simulink model "Wahadlo_final_2015a_2015a"  (R2019a)
settings: Solver=ode5  StartTime=0.0  StopTime=99999  FixedStep=0.01  RelTol=1e-3  AbsTol=1e-6
values from neighbouring files (symbols this model uses):
  K_later = [-K(1) -K(2) K(3)/3 K(4)/3]    [jacobian_calc.m]    (also in linearyzacja.m)
  k_soft_landing = 12    [init.m]
  K_stab = [-K(1) -K(2) K(3)/3 K(4)/3]    [jacobian_calc.m]    (also in linearyzacja.m)
  l = 0.2097    [init.m]    (also in linearyzacja.m = 0.107)
  relay = 0.4    [init.m]
undefined symbols (not defined in the file or in its folder): RTDAC4PCIBaseAddress, sigbuilder_block
settings Model: SimulationMode=external  ExtModeTrigDuration=60000  ExtModeTrigLevel=0.400000  Creator=jims  LastModifiedBy=Radosław
settings SolverCC: AutoScaleAbsTol=off
settings DataIOCC: ExternalInput=[]  InitialState=[]  MaxDataPoints=5000  SaveFormat=Array  SignalLoggingSaveFormat=ModelDataLogs  SaveOutput=off  SaveTime=off  ReturnWorkspaceOutputs=off  SignalLoggingName=sigsOut
settings OptimizationCC: BooleanDataType=off  ExpressionDepthLimit=2147483647  InitFltsAndDblsToZero=on  LifeSpan=inf
settings DebuggingCC: SaveWithParameterizedLinksMsg=none  UnderspecifiedInitializationDetection=Classic  MergeDetectMultiDrivingBlocksExec=none  SignalResolutionControl=TryResolveAllWithWarning  MultiTaskDSMMsg=warning  MultiTaskCondExecSysMsg=none  IntegerOverflowMsg=none  FcnCallInpInsideContextMsg=warning  StateNameClashWarn=warning  SFUnexpectedBacktrackingDiag=warning  SFNoUnconditionalDefaultTransitionDiag=warning  SFExecutionAtInitializationDiag=none  IntegerSaturationMsg=none  ArithmeticOperatorsInVariantConditions=warning
settings HardwareCC: ProdBitPerLong=64  ProdLargestAtomicFloat=None  ProdHWDeviceType=Intel->x86-64  TargetBitPerLong=64  TargetBitPerPointer=64  TargetIntDivRoundTo=Zero  TargetEndianess=LittleEndian  TargetWordSize=64  TargetHWDeviceType=Intel->x86-64
settings ModelReferenceCC: PropagateSignalLabelsOutOfModel=off
settings SFSimCC: SimUseLocalCustomCode=off
settings RTWCC: Description=Real-Time Windows Target  SystemTargetFile=rtwin.tlc  TemplateMakefile=RTDAC_win.tmf  RTWUseLocalCustomCode=off
settings CodeAppCC: StateflowObjectComments=on
settings TargetCC: TargetFcnLib=ansi_tfl_tmw.mat  TargetPreCompLibLocation=C:\Program Files\MATLAB\R2015aSP1\toolbox\sldrt\lib\win64  ModelReferenceCompliant=off  CompOptLevelCompliant=off  PreserveStateflowLocalDataDimensions=off
settings ConfigComp: CovMetricSettings=dw  CovHtmlReporting=on  CovSaveCumulativeToWorkspaceVar=on  CovSaveSingleToWorkspaceVar=on  CovExternalEMLEnable=off

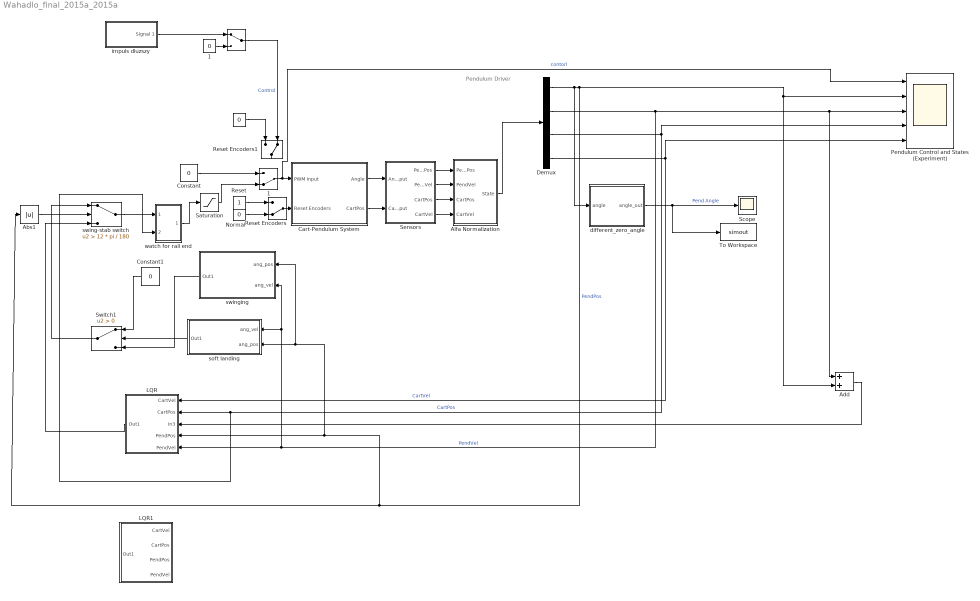
== system Wahadlo_final_2015a_2015a ==
  note: Pendulum
      | Driver
  " " : ManualSwitch
  " " : Constant  Value=0
  " 1" : Constant  Value=0
  " 1" : ManualSwitch  CurrentSetting=0
  Abs1 : Abs
  Add : Sum
  Alfa Normalization : Subsystem  mask(Choose mode:){pos=Inverted Pendulum}
      mask prompts: pos "Choose mode:"
      mask TypeOptions pos: Inverted Pendulum | Crane Controller
  Cart-Pendulum System : Subsystem  mask{BaseAddress=RTDAC4PCIBaseAddress(-1,-1), T0=0.01}
      mask prompts: BaseAddress "Base Address:"; T0 "Sampling Period:"
      mask Display: plot( [0.725 0.725], [1.05 0.375], 0.725+0.05*sin([0:0.5:7]), 0.325+0.05*cos([0:0.5:7]), [-0.3 -0.3], [-0.3 -0.3], [1.8 1.8], [1.8 1.8], [0.1 1.4], [0.95 0.95], [0.1 1.4], [0.92 0.92], [0.65 0.8], [1 1], [0.65 0.8], [1.1 1.1], [0.65 0.65], [1.1 1], [0.8 0.8], [1 1.1] )
  Constant : Constant  Value=0
  Constant1 : Constant  Value=0
  Demux : Demux
  LQR : Subsystem
  LQR1 : Subsystem
  Normal : Constant  Value=0
  Pendulum Control and States (Experiment) : Scope  NumInputPorts=5
  Reset : Constant
  Reset Encoders : ManualSwitch  CurrentSetting=0
  Reset Encoders1 : ManualSwitch  CurrentSetting=0
  Saturation : Saturate
  Scope : Scope
  Sensors : Subsystem  mask(PENDULUM Output){T0=0.01}
      mask prompts: T0 "Sample Time"
      mask help: PCL-812 PG Device Driver
  Switch1 : Switch  Criteria=u2 > Threshold
  To Workspace : ToWorkspace  VariableName=simout  SampleTime=-1
  "different_zero_angle " : MATLAB Function  TreatAsAtomicUnit=on
  "impuls dluzszy " : Subsystem  Tag=STV Subsys  LoadFcn=sigbuilder_block('load');  StartFcn=sigbuilder_block('start');  StopFcn=sigbuilder_block('stop');  ClipboardFcn=sigbuilder_block('clipboard');  mask(Sigbuilder block){tuvar=[0:10]}
      mask help: Simulink:masks:SigbuilderBlock_MD
      mask init:
      | if ~strcmp(get_param(bdroot(gcbh),'SimulationStatus'),'stopped') tuvar = sigbuilder_block('maskInit'); end
      settings: CopyFcn=sigbuilder_block('copy');  DeleteFcn=sigbuilder_block('delete');  ModelCloseFcn=sigbuilder_block('modelClose');  PreSaveFcn=sigbuilder_block('preSave');  PauseFcn=sigbuilder_block('pause');  ContinueFcn=sigbuilder_block('continue');  NameChangeFcn=sigbuilder_block('namechange');  OpenFcn=sigbuilder_block('open',[437.6 178.5 550.4 399.75 ]);  CloseFcn=sigbuilder_block('close');
      mask Display: plot(0, 0, 100, 100,[2, 2, 32, 32, 2], [68, 8, 8, 68, 68],[32, 2], [38, 38], [32, 19, 2],[53, 60, 44], [32, 17, 17, 2],[16, 16, 31, 31]);txt = getActiveGroup(gcbh);text(2, 100, txt,'verticalAlignment', 'top');
  "soft landing " : Subsystem
  "swing-stab switch " : Switch  Criteria=u2 > Threshold  Threshold=12 * pi / 180
  "swinging " : Subsystem
  watch for rail end : Subsystem
  wires:
  Reset Encoders/1 -> Cart-Pendulum System/2(Reset Encoders)
  Normal/1 -> Reset Encoders/2
  Reset/1 -> Reset Encoders/1
  Sensors/1(PendPos) -> Alfa Normalization/1(PendPos)
  Sensors/2(PendVel) -> Alfa Normalization/2(PendVel)
  Sensors/3(CartPos) -> Alfa Normalization/3(CartPos)
  Sensors/4(CartVel) -> Alfa Normalization/4(CartVel)
  Cart-Pendulum System/1(Angle) -> Sensors/1(AngleInput)
  Cart-Pendulum System/2(CartPos) -> Sensors/2(CartPosInput)
  Alfa Normalization/1(State) -> Demux/1
  Demux/4 -> Pendulum Control and States (Experiment)/5, LQR/1(CartVel)  "CartVel"
  Demux/3 -> LQR/2(CartPos), watch for rail end/2(cart pos), Pendulum Control and States (Experiment)/4  "CartPos"
  Demux/2 -> Add/1, Pendulum Control and States (Experiment)/3, "swinging "/2(ang_vel), "soft landing "/1("ang_vel "), LQR/5(PendVel)  "PendVel"
  Demux/1 -> "different_zero_angle "/1(angle), Abs1/1, "soft landing "/2("ang_pos "), "swinging "/1("ang_pos "), LQR/4(PendPos), Add/2, Pendulum Control and States (Experiment)/2  "PendPos"
  "different_zero_angle "/1(angle_out) -> To Workspace/1, Scope/1  "Pend Angle"
  " "/1 -> Reset Encoders1/2  "Control"
  " "/1 -> Reset Encoders1/1
  " 1"/1 -> " "/2
  "impuls dluzszy "/1(Signal 1) -> " "/1
  " 1"/1 -> Pendulum Control and States (Experiment)/1, Cart-Pendulum System/1(PWM Input)  "contorl"
  Constant/1 -> " 1"/1
  Constant1/1 -> Switch1/1
  "swinging "/1(Out1) -> Switch1/3
  "soft landing "/1(Out1) -> Switch1/2
  Abs1/1 -> "swing-stab switch "/2
  Saturation/1 -> " 1"/2
  watch for rail end/1(control_out) -> Saturation/1
  "swing-stab switch "/1 -> watch for rail end/1(control_in)
  Switch1/1 -> "swing-stab switch "/1
  Add/1 -> LQR/3(In3)
  LQR/1(Out1) -> "swing-stab switch "/3

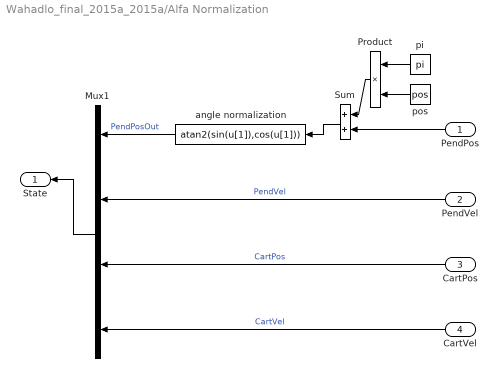
== system Wahadlo_final_2015a_2015a/Alfa Normalization ==
  PendPos : Inport
  PendVel : Inport  Port=2
  CartPos : Inport  Port=3
  CartVel : Inport  Port=4
  Mux1 : Mux
  Product : Product  SaturateOnIntegerOverflow=on  InputSameDT=on  OutDataTypeStr=Inherit: Same as first input
  Sum : Sum  SaturateOnIntegerOverflow=on  InputSameDT=on  OutDataTypeStr=Inherit: Same as first input
  angle normalization : Fcn  Expr=atan2(sin(u[1]),cos(u[1]))
  pi : Constant  Value=pi
  pos : Constant  Value=pos
  State : Outport  InitialOutput=0  VectorParamsAs1DForOutWhenUnconnected=off
  wires:
  angle normalization/1 -> Mux1/1  "PendPosOut"
  PendVel/1 -> Mux1/2  "PendVel"
  CartVel/1 -> Mux1/4  "CartVel"
  CartPos/1 -> Mux1/3  "CartPos"
  Mux1/1 -> State/1
  Sum/1 -> angle normalization/1
  PendPos/1 -> Sum/2
  pi/1 -> Product/1
  pos/1 -> Product/2
  Product/1 -> Sum/1

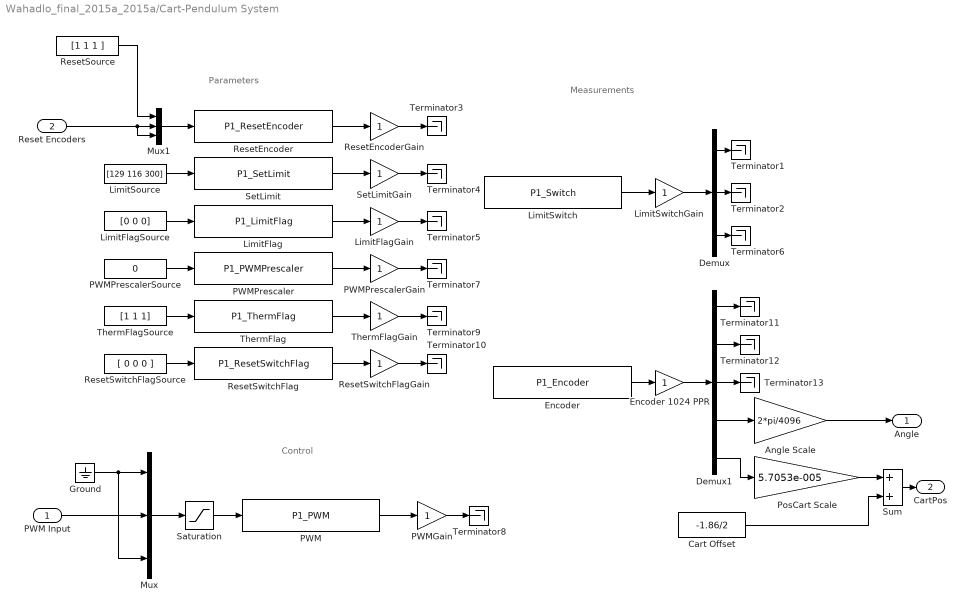
== system Wahadlo_final_2015a_2015a/Cart-Pendulum System ==
  note: Measurements
  note: Control
  note: Parameters
  PWM Input : Inport
  Reset Encoders : Inport  Port=2
  Angle Scale : Gain  Gain=2*pi/4096  OutDataTypeStr=Inherit: Same as input  ParamDataTypeStr=Inherit: Same as input
  Cart Offset : Constant  Value=-1.86/2
  Demux : Demux  Outputs=3
  Demux1 : Demux  Outputs=5
  Encoder : S-Function  FunctionName=P1_Encoder  Parameters=BaseAddress, T0  SFunctionDeploymentMode=off  EnableBusSupport=off
  Encoder 1024 PPR : Gain  SaturateOnIntegerOverflow=on  OutDataTypeStr=Inherit: Same as input  ParamDataTypeStr=Inherit: Same as input
  Ground : Ground
  LimitFlag : S-Function  FunctionName=P1_LimitFlag  Parameters=BaseAddress, T0  SFunctionDeploymentMode=off  EnableBusSupport=off
  LimitFlagGain : Gain  SaturateOnIntegerOverflow=on  OutDataTypeStr=Inherit: Same as input  ParamDataTypeStr=Inherit: Same as input
  LimitFlagSource : Constant  Value=[0 0 0]
  LimitSource : Constant  Value=[129 116 300]
  LimitSwitch : S-Function  FunctionName=P1_Switch  Parameters=BaseAddress, T0  SFunctionDeploymentMode=off  EnableBusSupport=off
  LimitSwitchGain : Gain  SaturateOnIntegerOverflow=on  OutDataTypeStr=Inherit: Same as input  ParamDataTypeStr=Inherit: Same as input
  Mux : Mux  Inputs=3
  Mux1 : Mux  Inputs=[3 1 1]
  PWM : S-Function  FunctionName=P1_PWM  Parameters=BaseAddress, T0  SFunctionDeploymentMode=off  EnableBusSupport=off
  PWMGain : Gain  SaturateOnIntegerOverflow=on  OutDataTypeStr=Inherit: Same as input  ParamDataTypeStr=Inherit: Same as input
  PWMPrescaler : S-Function  FunctionName=P1_PWMPrescaler  Parameters=BaseAddress, T0  SFunctionDeploymentMode=off  EnableBusSupport=off
  PWMPrescalerGain : Gain  SaturateOnIntegerOverflow=on  OutDataTypeStr=Inherit: Same as input  ParamDataTypeStr=Inherit: Same as input
  PWMPrescalerSource : Constant  Value=0
  PosCart Scale : Gain  Gain=5.7053e-005  OutDataTypeStr=Inherit: Same as input  ParamDataTypeStr=Inherit: Same as input
  ResetEncoder : S-Function  FunctionName=P1_ResetEncoder  Parameters=BaseAddress, T0  SFunctionDeploymentMode=off  EnableBusSupport=off
  ResetEncoderGain : Gain  SaturateOnIntegerOverflow=on  OutDataTypeStr=Inherit: Same as input  ParamDataTypeStr=Inherit: Same as input
  ResetSource : Constant  Value=[1 1 1 ]
  "ResetSwitchFlag " : S-Function  FunctionName=P1_ResetSwitchFlag  Parameters=BaseAddress, T0  SFunctionDeploymentMode=off  EnableBusSupport=off
  ResetSwitchFlagGain : Gain  SaturateOnIntegerOverflow=on  OutDataTypeStr=Inherit: Same as input  ParamDataTypeStr=Inherit: Same as input
  ResetSwitchFlagSource : Constant  Value=[ 0 0 0 ]
  Saturation : Saturate
  SetLimit : S-Function  FunctionName=P1_SetLimit  Parameters=BaseAddress, T0  SFunctionDeploymentMode=off  EnableBusSupport=off
  SetLimitGain : Gain  SaturateOnIntegerOverflow=on  OutDataTypeStr=Inherit: Same as input  ParamDataTypeStr=Inherit: Same as input
  Sum : Sum  SaturateOnIntegerOverflow=on  InputSameDT=on  OutDataTypeStr=Inherit: Same as first input
  Terminator{1..13} (13 alike) : Terminator
  "ThermFlag " : S-Function  FunctionName=P1_ThermFlag  Parameters=BaseAddress, T0  SFunctionDeploymentMode=off  EnableBusSupport=off
  ThermFlagGain : Gain  SaturateOnIntegerOverflow=on  OutDataTypeStr=Inherit: Same as input  ParamDataTypeStr=Inherit: Same as input
  ThermFlagSource : Constant  Value=[1 1 1]
  Angle : Outport  VectorParamsAs1DForOutWhenUnconnected=off
  CartPos : Outport  Port=2  VectorParamsAs1DForOutWhenUnconnected=off
  wires:
  Demux1/1 -> Terminator11/1
  Demux1/2 -> Terminator12/1
  Demux1/3 -> Terminator13/1
  Demux1/4 -> Angle Scale/1
  Demux1/5 -> PosCart Scale/1
  Angle Scale/1 -> Angle/1
  Demux/3 -> Terminator6/1
  Demux/2 -> Terminator2/1
  Demux/1 -> Terminator1/1
  LimitSwitchGain/1 -> Demux/1
  LimitSwitch/1 -> LimitSwitchGain/1
  Ground/1 -> Mux/1, Mux/3
  PWM Input/1 -> Mux/2
  ResetSwitchFlagGain/1 -> Terminator10/1
  ThermFlagGain/1 -> Terminator9/1
  PWMPrescalerGain/1 -> Terminator7/1
  LimitFlagGain/1 -> Terminator5/1
  SetLimitGain/1 -> Terminator4/1
  ResetEncoderGain/1 -> Terminator3/1
  ResetSwitchFlagSource/1 -> "ResetSwitchFlag "/1
  ThermFlagSource/1 -> "ThermFlag "/1
  PWMPrescalerSource/1 -> PWMPrescaler/1
  LimitFlagSource/1 -> LimitFlag/1
  LimitSource/1 -> SetLimit/1
  "ResetSwitchFlag "/1 -> ResetSwitchFlagGain/1
  "ThermFlag "/1 -> ThermFlagGain/1
  PWMPrescaler/1 -> PWMPrescalerGain/1
  LimitFlag/1 -> LimitFlagGain/1
  SetLimit/1 -> SetLimitGain/1
  ResetEncoder/1 -> ResetEncoderGain/1
  PWMGain/1 -> Terminator8/1
  PWM/1 -> PWMGain/1
  Mux/1 -> Saturation/1
  Saturation/1 -> PWM/1
  Encoder/1 -> Encoder 1024 PPR/1
  Encoder 1024 PPR/1 -> Demux1/1
  Mux1/1 -> ResetEncoder/1
  ResetSource/1 -> Mux1/1
  Reset Encoders/1 -> Mux1/2, Mux1/3
  PosCart Scale/1 -> Sum/1
  Sum/1 -> CartPos/1
  Cart Offset/1 -> Sum/2

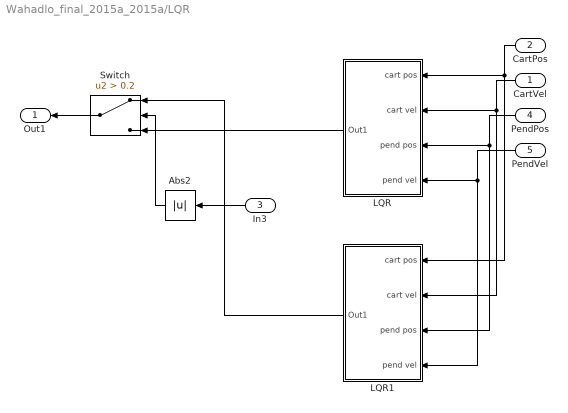
== system Wahadlo_final_2015a_2015a/LQR ==
  CartVel : Inport
  CartPos : Inport  Port=2
  In3 : Inport  Port=3
  PendPos : Inport  Port=4
  PendVel : Inport  Port=5
  Abs2 : Abs
  LQR : Subsystem
  LQR1 : Subsystem
  Switch : Switch  Criteria=u2 > Threshold  Threshold=0.2
  Out1 : Outport  VectorParamsAs1DForOutWhenUnconnected=off
  wires:
  LQR1/1(Out1) -> Switch/1
  LQR/1(Out1) -> Switch/3
  In3/1 -> Abs2/1
  PendVel/1 -> LQR1/4("pend vel "), LQR/4("pend vel ")
  CartPos/1 -> LQR/1(cart pos), LQR1/1(cart pos)
  PendPos/1 -> LQR1/3(pend pos), LQR/3(pend pos)
  Abs2/1 -> Switch/2
  Switch/1 -> Out1/1
  CartVel/1 -> LQR1/2("cart vel "), LQR/2("cart vel ")

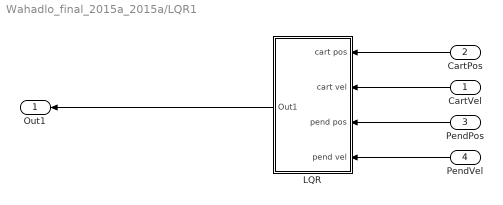
== system Wahadlo_final_2015a_2015a/LQR1 ==
  CartVel : Inport
  CartPos : Inport  Port=2
  PendPos : Inport  Port=3
  PendVel : Inport  Port=4
  LQR : Subsystem
  Out1 : Outport  VectorParamsAs1DForOutWhenUnconnected=off
  wires:
  PendVel/1 -> LQR/4("pend vel ")
  CartPos/1 -> LQR/1(cart pos)
  PendPos/1 -> LQR/3(pend pos)
  LQR/1(Out1) -> Out1/1
  CartVel/1 -> LQR/2("cart vel ")

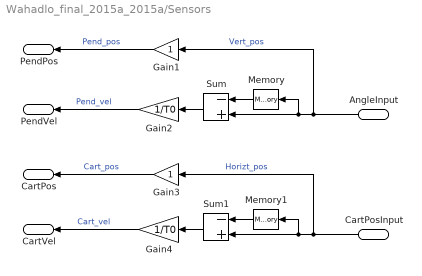
== system Wahadlo_final_2015a_2015a/Sensors ==
  AngleInput : Inport
  CartPosInput : Inport  Port=2
  Gain1 : Gain  SaturateOnIntegerOverflow=on  OutDataTypeStr=Inherit: Same as input  ParamDataTypeStr=Inherit: Same as input
  Gain2 : Gain  Gain=1/T0  SaturateOnIntegerOverflow=on  OutDataTypeStr=Inherit: Same as input  ParamDataTypeStr=Inherit: Same as input
  Gain3 : Gain  SaturateOnIntegerOverflow=on  OutDataTypeStr=Inherit: Same as input  ParamDataTypeStr=Inherit: Same as input
  Gain4 : Gain  Gain=1/T0  SaturateOnIntegerOverflow=on  OutDataTypeStr=Inherit: Same as input  ParamDataTypeStr=Inherit: Same as input
  Memory : Memory
  Memory1 : Memory
  Sum : Sum  Inputs=-+  SaturateOnIntegerOverflow=on  InputSameDT=on  OutDataTypeStr=Inherit: Same as first input
  Sum1 : Sum  Inputs=-+  SaturateOnIntegerOverflow=on  InputSameDT=on  OutDataTypeStr=Inherit: Same as first input
  PendPos : Outport  InitialOutput=0  VectorParamsAs1DForOutWhenUnconnected=off
  PendVel : Outport  Port=2  InitialOutput=0  VectorParamsAs1DForOutWhenUnconnected=off
  CartPos : Outport  Port=3  InitialOutput=0  VectorParamsAs1DForOutWhenUnconnected=off
  CartVel : Outport  Port=4  InitialOutput=0  VectorParamsAs1DForOutWhenUnconnected=off
  wires:
  Gain4/1 -> CartVel/1  "Cart_vel"
  Sum1/1 -> Gain4/1
  Memory1/1 -> Sum1/1
  Sum/1 -> Gain2/1
  Memory/1 -> Sum/1
  CartPosInput/1 -> Memory1/1, Sum1/2, Gain3/1  "Horizt_pos"
  AngleInput/1 -> Memory/1, Sum/2, Gain1/1  "Vert_pos"
  Gain2/1 -> PendVel/1  "Pend_vel"
  Gain1/1 -> PendPos/1  "Pend_pos"
  Gain3/1 -> CartPos/1  "Cart_pos"

== system Wahadlo_final_2015a_2015a/impuls dluzszy  ==
  Demux : Demux  Tag=STV Demux  Outputs=1
  FromWs : FromWorkspace  Tag=STV FromWs  VariableName=tuvar  SampleTime=0
      SigBuilderData=|
      | common.afterFinalStr = 'Extrapolate'
      | common.sampleTime = 0
      | dataSet.timeRange = [0 10]
      | dataSet.name = 'Group 1'
      | sbobj.Groups.Name = 'Group 1'
      | sbobj.Groups.Signals.Name = 'Signal 1'
      | sbobj.Groups.Signals.XData = [0 1.2 1.2 1.8 1.8 2.3 2.3 10]
      | sbobj.Groups.Signals.YData = [0 0 -0.5 -0.5 0.5 0.5 0 -7.08027892008e-05]
  Signal 1 : Outport  Tag=STV Outport  VectorParamsAs1DForOutWhenUnconnected=off
  wires:
  Demux/1 -> Signal 1/1
  FromWs/1 -> Demux/1

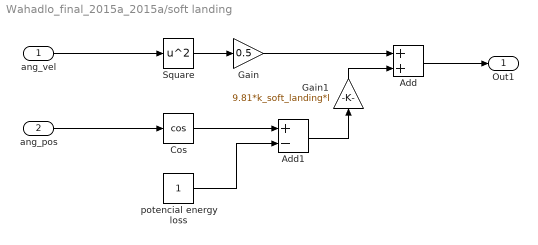
== system Wahadlo_final_2015a_2015a/soft landing  ==
  "ang_vel " : Inport
  "ang_pos " : Inport  Port=2
  Add : Sum
  Add1 : Sum  Inputs=+-
  Cos : Trigonometry  Operator=cos
  Gain : Gain  Gain=0.5
  Gain1 : Gain  Gain=9.81*k_soft_landing*l
  Square : Math  Operator=square  SaturateOnIntegerOverflow=on
  "potencial energy loss " : Constant
  Out1 : Outport  VectorParamsAs1DForOutWhenUnconnected=off
  wires:
  Square/1 -> Gain/1
  Gain/1 -> Add/1
  Cos/1 -> Add1/1
  "potencial energy loss "/1 -> Add1/2
  Add/1 -> Out1/1
  "ang_pos "/1 -> Cos/1
  "ang_vel "/1 -> Square/1
  Gain1/1 -> Add/2
  Add1/1 -> Gain1/1

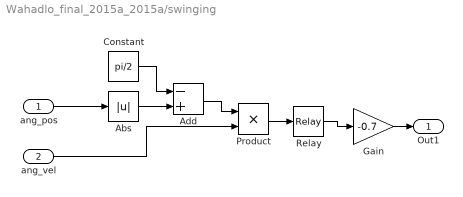
== system Wahadlo_final_2015a_2015a/swinging  ==
  "ang_pos " : Inport
  ang_vel : Inport  Port=2
  Abs : Abs
  Add : Sum  Inputs=-+
  Constant : Constant  Value=pi/2
  Gain : Gain  Gain=-0.7
  Product : Product
  Relay : Relay  OnSwitchValue=relay  OffSwitchValue=-relay  OnOutputValue=0.5  OffOutputValue=-0.5
  Out1 : Outport  VectorParamsAs1DForOutWhenUnconnected=off
  wires:
  ang_vel/1 -> Product/2
  "ang_pos "/1 -> Abs/1
  Abs/1 -> Add/2
  Add/1 -> Product/1
  Constant/1 -> Add/1
  Product/1 -> Relay/1
  Relay/1 -> Gain/1
  Gain/1 -> Out1/1

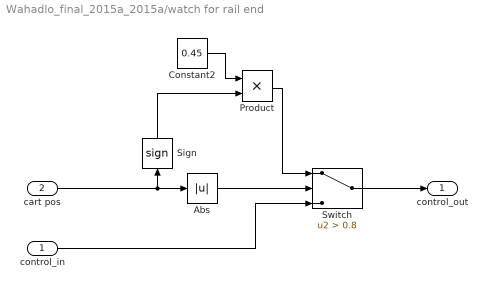
== system Wahadlo_final_2015a_2015a/watch for rail end ==
  control_in : Inport
  cart pos : Inport  Port=2
  Abs : Abs
  Constant2 : Constant  Value=0.45
  Product : Product
  Sign : Signum
  Switch : Switch  Criteria=u2 > Threshold  Threshold=0.8
  control_out : Outport  VectorParamsAs1DForOutWhenUnconnected=off
  wires:
  Switch/1 -> control_out/1
  cart pos/1 -> Sign/1, Abs/1
  Abs/1 -> Switch/2
  Constant2/1 -> Product/1
  Sign/1 -> Product/2
  control_in/1 -> Switch/3
  Product/1 -> Switch/1

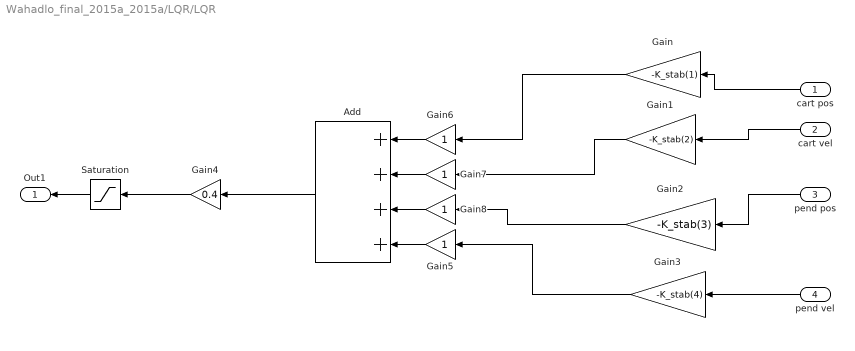
== system Wahadlo_final_2015a_2015a/LQR/LQR ==
  cart pos : Inport
  "cart vel " : Inport  Port=2
  pend pos : Inport  Port=3
  "pend vel " : Inport  Port=4
  Add : Sum  Inputs=++++
  Gain : Gain  Gain=-K_stab(1)
  Gain1 : Gain  Gain=-K_stab(2)
  Gain2 : Gain  Gain=-K_stab(3)
  Gain3 : Gain  Gain=-K_stab(4)
  Gain4 : Gain  Gain=0.4
  Gain{5..8} (4 alike) : Gain
  Saturation : Saturate
  Out1 : Outport  VectorParamsAs1DForOutWhenUnconnected=off
  wires:
  pend pos/1 -> Gain2/1
  "cart vel "/1 -> Gain1/1
  "pend vel "/1 -> Gain3/1
  cart pos/1 -> Gain/1
  Gain/1 -> Gain6/1
  Gain1/1 -> Gain7/1
  Gain2/1 -> Gain8/1
  Gain3/1 -> Gain5/1
  Saturation/1 -> Out1/1
  Add/1 -> Gain4/1
  Gain4/1 -> Saturation/1
  Gain5/1 -> Add/4
  Gain8/1 -> Add/3
  Gain7/1 -> Add/2
  Gain6/1 -> Add/1

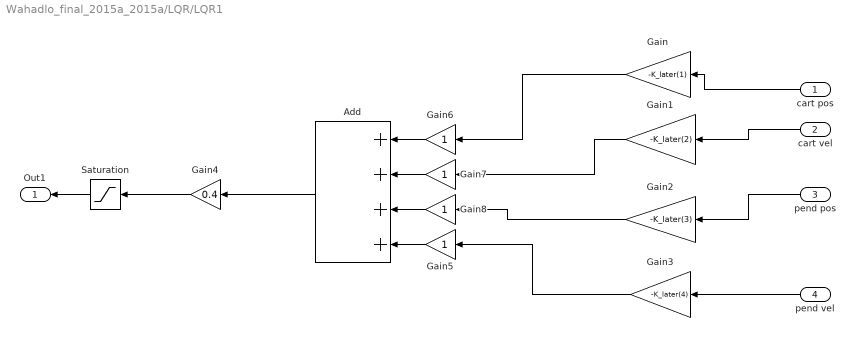
== system Wahadlo_final_2015a_2015a/LQR/LQR1 ==
  cart pos : Inport
  "cart vel " : Inport  Port=2
  pend pos : Inport  Port=3
  "pend vel " : Inport  Port=4
  Add : Sum  Inputs=++++
  Gain : Gain  Gain=-K_later(1)
  Gain1 : Gain  Gain=-K_later(2)
  Gain2 : Gain  Gain=-K_later(3)
  Gain3 : Gain  Gain=-K_later(4)
  Gain4 : Gain  Gain=0.4
  Gain{5..8} (4 alike) : Gain
  Saturation : Saturate
  Out1 : Outport  VectorParamsAs1DForOutWhenUnconnected=off
  wires:
  pend pos/1 -> Gain2/1
  "cart vel "/1 -> Gain1/1
  "pend vel "/1 -> Gain3/1
  cart pos/1 -> Gain/1
  Gain/1 -> Gain6/1
  Gain1/1 -> Gain7/1
  Gain2/1 -> Gain8/1
  Gain3/1 -> Gain5/1
  Saturation/1 -> Out1/1
  Add/1 -> Gain4/1
  Gain4/1 -> Saturation/1
  Gain5/1 -> Add/4
  Gain8/1 -> Add/3
  Gain7/1 -> Add/2
  Gain6/1 -> Add/1

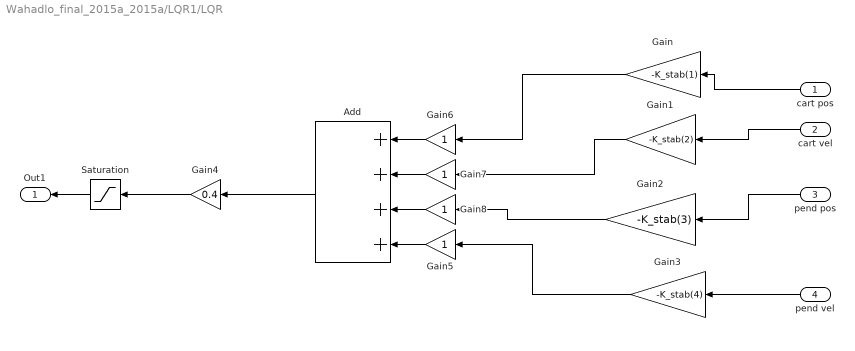
== system Wahadlo_final_2015a_2015a/LQR1/LQR ==
  cart pos : Inport
  "cart vel " : Inport  Port=2
  pend pos : Inport  Port=3
  "pend vel " : Inport  Port=4
  Add : Sum  Inputs=++++
  Gain : Gain  Gain=-K_stab(1)
  Gain1 : Gain  Gain=-K_stab(2)
  Gain2 : Gain  Gain=-K_stab(3)
  Gain3 : Gain  Gain=-K_stab(4)
  Gain4 : Gain  Gain=0.4
  Gain{5..8} (4 alike) : Gain
  Saturation : Saturate
  Out1 : Outport  VectorParamsAs1DForOutWhenUnconnected=off
  wires:
  pend pos/1 -> Gain2/1
  "cart vel "/1 -> Gain1/1
  "pend vel "/1 -> Gain3/1
  cart pos/1 -> Gain/1
  Gain/1 -> Gain6/1
  Gain1/1 -> Gain7/1
  Gain2/1 -> Gain8/1
  Gain3/1 -> Gain5/1
  Saturation/1 -> Out1/1
  Add/1 -> Gain4/1
  Gain4/1 -> Saturation/1
  Gain5/1 -> Add/4
  Gain8/1 -> Add/3
  Gain7/1 -> Add/2
  Gain6/1 -> Add/1

== matlab function Wahadlo_final_2015a_2015a/different_zero_angle  ==
  data: angle input; angle_out output
function angle_out = fcn(angle)

if(angle > 0)
    angle = angle - pi;
elseif(angle == 0)
    angle = angle;
else
    angle = angle + pi;
end
angle_out = angle * 180 / pi
